simulink model "can_bus"  (R2023b)
settings: Solver=VariableStepAuto  StartTime=0.0  StopTime=inf  RelTol=1e-3
undefined symbols (not defined in the file): canChannel
libraries: canlib x3, canmsglib x2
settings Model: LastModifiedBy=huyang

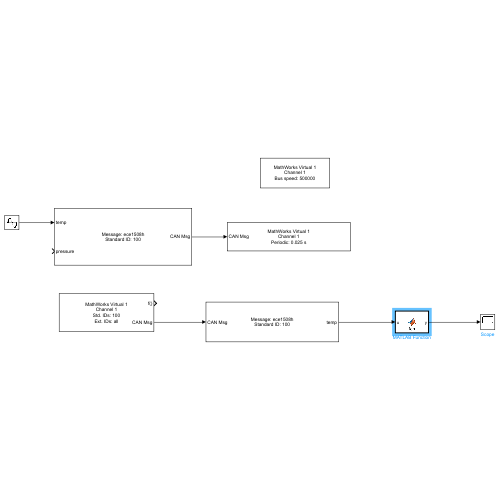
[thumbnail: Simulink's stored preview of the top-level diagram]
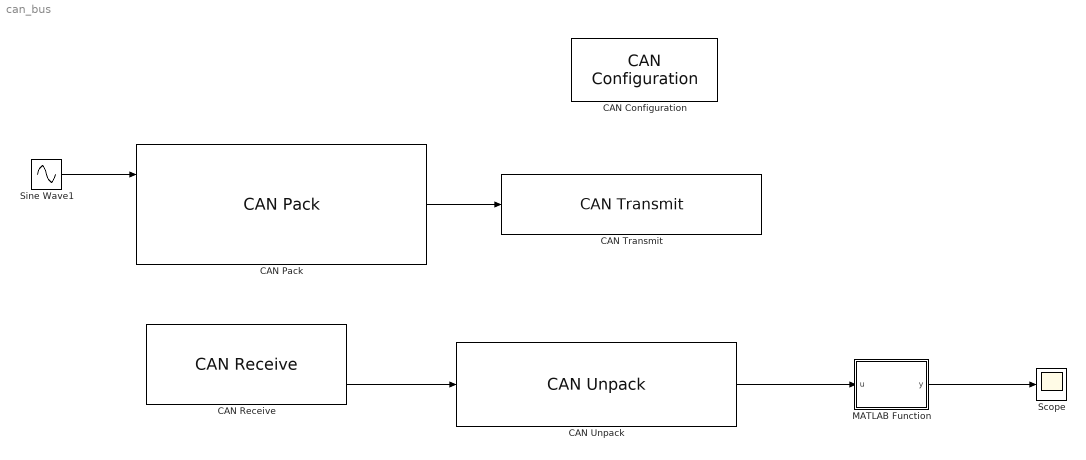
== system can_bus ==
  CAN Configuration : canlib/CAN Configuration  BlockHandle=246.0002  Device=MathWorks Virtual 1 (Channel 1)  DeviceMenu=MathWorks Virtual 1 (Channel 1)  ObjConstructor=canChannel('MathWorks', 'Virtual 1', 1)  BusSpeed=500000  EnableBitParameters=off  AckMode=Normal
  CAN Pack : canmsglib/CAN Pack  MsgList=(none)  MsgName=ece1508h  MsgIDType=Standard (11-bit identifier)  MsgIdentifier=100  MsgLength=8  Remote=off  ApplyMinMax=off  BusOutput=off  SignalInfo={ 'temp', '0', '8', 'LE', 'signed', 'Standard', '0', '1', '0', '-Inf', 'Inf'; 'pressure', '8', '8', 'LE', 'signed', 'Standard', '0', '1', '0', '-Inf', 'Inf' }
      settings: LibrarySourceBlock=canlib/CAN Pack  DataFormat=manually specified signals
  CAN Receive : canlib/CAN Receive  BlockHandle=248.0002  Device=MathWorks Virtual 1 (Channel 1)  DeviceMenu=MathWorks Virtual 1 (Channel 1)  ObjConstructor=canChannel('MathWorks', 'Virtual 1', 1)  EnableStandardIDsFilter=off  StdIDsCombo=Allow only  StandardIDs=100  EnableExtendedIDsFilter=off  ExtIDsCombo=Allow all  ExtendedIDs=0  SampleTime=0.00001  MsgsPerTimestep=all  InternalFilterUpdateStatus=on  BusOutput=off
  CAN Transmit : canlib/CAN Transmit  BlockHandle=249.0002  Device=MathWorks Virtual 1 (Channel 1)  DeviceMenu=MathWorks Virtual 1 (Channel 1)  ObjConstructor=canChannel('MathWorks', 'Virtual 1', 1)  EnableEventTransmit=off  EnablePeriodicTransmit=on  MessagePeriod=0.025
  CAN Unpack : canmsglib/CAN Unpack  MsgList=(none)  MsgName=ece1508h  MsgIDType=Standard (11-bit identifier)  MsgIdentifier=100  MsgLength=8  SignalInfo={ 'temp', '0', '8', 'LE', 'signed', 'Standard', '0', '1', '0', '-Inf', 'Inf' }  IDPort=off  TimestampPort=off  ErrorPort=off  RemotePort=off  LengthPort=off  StatusPort=off  ApplyMinMax=off
      settings: LibrarySourceBlock=canlib/CAN Unpack
  MATLAB Function : MATLAB Function  TreatAsAtomicUnit=on
  Scope : Scope
  Sine Wave1 : Sin  SampleTime=0.001
  wires:
  Sine Wave1/1 -> CAN Pack/1
  CAN Pack/1 -> CAN Transmit/1
  CAN Receive/2 -> CAN Unpack/1
  CAN Unpack/1 -> MATLAB Function/1(u)
  MATLAB Function/1(y) -> Scope/1

== matlab function can_bus/MATLAB Function ==
  data: u input; y output
function y = fcn(u)

% TODO: implement intrusion detection algorithm here

y = u;
